simulink subsystem "AC_Source_with_Linear_droopControl"  (R2021a)
settings: Solver=VariableStepAuto  StartTime=0.0  StopTime=10.0  RelTol=1e-3
libraries: spsControlledCurrentSourceLib x1, spsControlledVoltageSourceLib x1
settings Model: Creator=FAST  LastModifiedBy=Sajid Ali

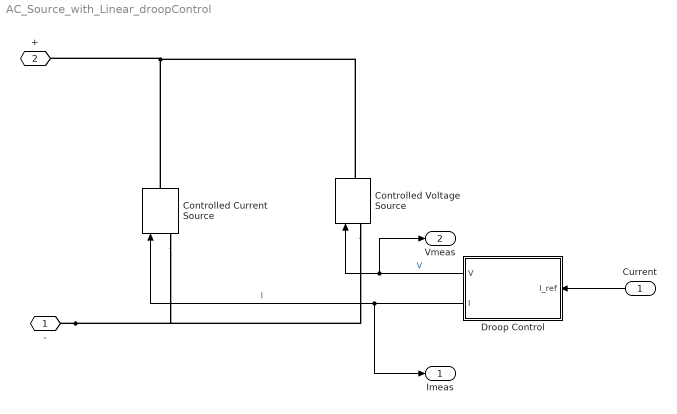
== system AC_Source_with_Linear_droopControl ==
  Current : Inport
  Controlled Current Source : spsControlledCurrentSourceLib/Controlled Current Source  Initialize=on  Source_Type=AC  Amplitude=0  Phase=0  Frequency=0  Measurements=None
  Controlled Voltage Source : spsControlledVoltageSourceLib/Controlled Voltage Source  Initialize=on  Source_Type=AC  Amplitude=0  Phase=0  Frequency=0  Measurements=None
  Droop Control : Subsystem  mask{Irated=10, Vnom=120, Vrated=100}
      mask prompts: Irated "Maximum Current (A)"; Vnom "Maximum Voltage (V)"; Vrated "Minimum Voltage (V)"
      mask init:
      | m=(Vnom-Vrated)/Irated;
      mask DialogControl DescGroupVar Prompt: Description about the block
      mask DialogControl DescTextVar Prompt: This block implements a linear droop control with saturation limit on input current Author:sajidali
  - : PMIOPort  Side=Left
  + : PMIOPort  Port=2  Side=Right
  Imeas : Outport
  Vmeas : Outport  Port=2
  wires:
  Current/1 -> Droop Control/1(I_ref)
  Droop Control/2(I) -> Controlled Current Source/1, Imeas/1  "I"
  Droop Control/1(V) -> Controlled Voltage Source/1, Vmeas/1  "V"
  connections:
  Controlled Voltage Source/RConn1 -- +/RConn1 -- Controlled Current Source/RConn1
  -/RConn1 -- Controlled Voltage Source/LConn1 -- Controlled Current Source/LConn1

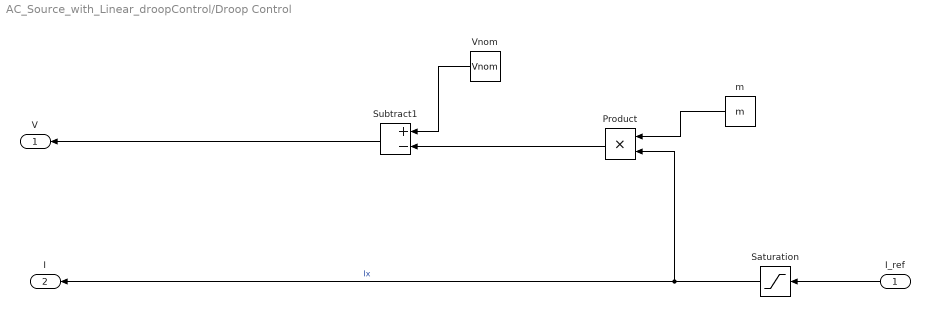
== system AC_Source_with_Linear_droopControl/Droop Control ==
  I_ref : Inport
  Product : Product
  Saturation : Saturate  UpperLimit=Irated  LowerLimit=0
  Subtract1 : Sum  Inputs=+-
  Vnom : Constant  Value=Vnom
  m : Constant  Value=m
  V : Outport
  I : Outport  Port=2
  wires:
  I_ref/1 -> Saturation/1
  Subtract1/1 -> V/1
  Saturation/1 -> Product/2, I/1  "Ix"
  m/1 -> Product/1
  Vnom/1 -> Subtract1/1
  Product/1 -> Subtract1/2
